simulink model "VFD3"  (R2020a)
settings: Solver=VariableStepAuto  StartTime=0.0  StopTime=100  RelTol=0.5e-3
libraries: fl_lib x51, nesl_utility x29, ee_lib x15, powerlib_meascontrol x2
settings Model: Creator=WASHINGTON  LastModifiedBy=WASHINGTON
settings SolverCC: MaxConsecutiveMinStep=100  AlgebraicLoopSolver=LineSearch

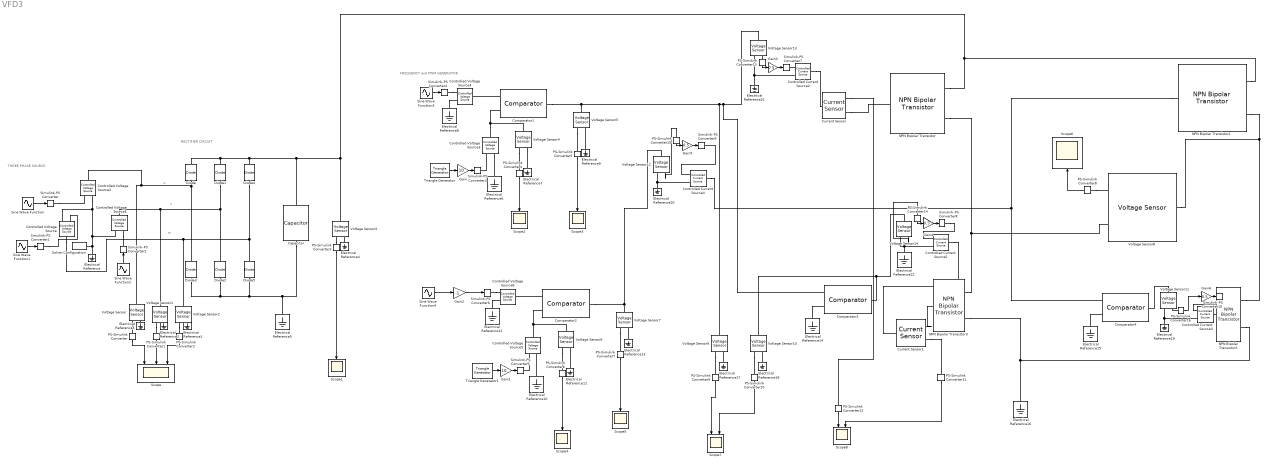
== system VFD3 ==
  note: FREQUENCY and PWM GENERATOR
  note: RECTIFIER CIRCUIT
  note: w
  note: v
  note: u
  note: THREE PHASE SOURCE
  Capacitor : ee_lib/Passive/Capacitor  cap_option=0  c=1 mF  Cvec=[1e-05, 1e-06] F  Vvec=[0, 10] V  CV_table_symmetry=1  f_vec=[1, 10] kHz  DFext_vec=[.8, 1.2]  C_tol=5  enable_C_tol=0  tol_distribution=1  nSigma=4  r=1e-6 Ohm  g=0 1/Ohm  averaging_period=0 s  enable_operating_limits=0  operating_limit_action=2  max_working_voltage_range=[-25, 25] V  power_rating=1 W  enable_faults=0  fault_action=1  Cscale_faulted=100  R_faulted=1e-3 Ohm  G_faulted=0 1/Ohm  tau_fault=1e-3 s  enable_temporal_fault=0  t_fault=1 s  enable_behavioral_fault=0  max_permissible_voltage_range=[-100, 100] V  t_fail_on_voltage=1 s  i_specify=off  i_priority=None  i=0 A  i_nominal_specify=off  i_nominal_unit=A  i_nominal_value=1  v_specify=off  v_priority=None  v=0 V  v_nominal_specify=off  v_nominal_unit=V  v_nominal_value=1  vc_specify=off  vc_priority=High  vc=0 V  vc_nominal_specify=off  vc_nominal_unit=V  vc_nominal_value=1
  Comparator{1..4} (4 alike) : ee_lib/Integrated Circuits/Comparator  V_OS=5 mV  V_OL=0 V  V_OH=10 V  C_IN=0 pF  R_OUT=50 Ohm  Delay=0 s
      settings: SourceProductBaseCode=PS  InternalSimscapePortConfiguration="{\"Bottom\":[],\"Left\":[{\"id\":\"p\",\"label\":\"+\",\"type\":\"foundation.electrical.electrical\"},{\"id\":\"n\",\"label\":\"-\",\"type\":\"foundation.electrical.electrical\"}],\"Right\":[{\"id\":\"J\",\"label\":\"\",\"type\":\"foundation.electrical.electrical\"}],\"Top\":[]}"
  Controlled Current Source{2..5} (4 alike) : fl_lib/Electrical/Electrical Sources/Controlled Current Source
  Controlled Voltage Source{,1..6} (7 alike) : fl_lib/Electrical/Electrical Sources/Controlled Voltage Source
  Current Sensor : fl_lib/Electrical/Electrical Sensors/Current Sensor
  Current Sensor1 : fl_lib/Electrical/Electrical Sensors/Current Sensor
  Diode{,1..5} (6 alike) : ee_lib/Semiconductors & Converters/Diode  ModelType=ee.enum.diode.modelType.pwl  Vf=0.6 V  Ron=0.3 Ohm  Goff=1e-8 S  prmExp=ee.enum.diode.expParam.useTwo  I12=[.0137, .545] A  V12=[.6, .7] V  IS=1e-12 A  ec=1  I1=0.0137 A  V1=0.6 V  RS=0 Ohm  Tmeas=25 degC  N_series=1  N_parallel=1  Rz=0.3 Ohm  BV=inf V  C_param=ee.enum.diode.capParam.fixed  CJ=5 pF  CJ0=5 pF  VJ=1 V  Mgrad=0.5  Vvec=[.1, 10, 100] V  Cvec=[3.5, 1, .4] pF  FC=0.5  Q_param=ee.enum.diode.recoveryParam.off  iRM=-7.15 A  iF=4 A  didt=-750 A/us  trr_factor=3  trr=115 ns  Qrr=1500 s*uA  TT=50 ns  tau=100 ns  T_param=ee.enum.diode.temperatureParam.off  IS_T2=1.25e-7 A  I1_T2=0.245 A  V1_T2=0.5 V  Tmeas2=125 degC  EG_param=ee.enum.diode.egapParam.material_si  EG=1.11 eV  XTI_param=ee.enum.diode.xtiParam.pn  XTI=3  dBVdT=0 V/K  Tdevice=25 degC  i_specify=off  i_priority=None  i=0 A  i_nominal_specify=off  i_nominal_unit=A  i_nominal_value=1  v_specify=off  v_priority=None  v=0 V  v_nominal_specify=off  v_nominal_unit=V  v_nominal_value=1  i_capacitor_specify=off  i_capacitor_priority=None  i_capacitor=0 A  i_capacitor_nominal_specify=off  i_capacitor_nominal_unit=A  i_capacitor_nominal_value=1  v_capacitor_specify=off  v_capacitor_priority=None  v_capacitor=0 V  v_capacitor_nominal_specify=off  v_capacitor_nominal_unit=V  v_capacitor_nominal_value=1  power_dissipated_specify=off  power_dissipated_priority=None  power_dissipated=0 W  power_dissipated_nominal_specify=off  power_dissipated_nominal_unit=W  power_dissipated_nominal_value=1  thermal_network_parameterization=ee.enum.thermalNetworkTopology.cauer  Rth=[0, 10] K/W  Rth_Foster=[4, 6] K/W  thermal_mass_parameterization=ee.enum.thermalNetwork.timeconstant  thermal_mass=[0, 1] J/K  thermal_mass_Foster=[1.5, 3] J/K  thermal_time_constant=[0, 10] s  thermal_time_constant_Foster=[6, 18] s  thermal_mass_initial_temperatures=[25, 25] degC
  Electrical Reference{,1..22} (23 alike) : fl_lib/Electrical/Electrical Elements/Electrical Reference
      settings: SourceProductBaseCode=MT,SS
  Gain : Gain  Gain=10
  Gain1 : Gain  Gain=10
  Gain2 : Gain  Gain=-1
  Gain{3..6} (4 alike) : Gain  Gain=0.5
  NPN Bipolar Transistor{,1..3} (4 alike) : ee_lib/Semiconductors & Converters/NPN Bipolar Transistor  parameterization=1  prmDatasheet=1  prmEquCoeff=1  BF=100  IS=1e-14 A  VAF=200 V  hfe=100  hoe=50e-6 1/Ohm  Ic_h=1 mA  Vce_h=5 V  V1=0.55 V  I1=0.5 mA  BR=1  Tmeas=25 degC  RC=0.01 Ohm  RE=1e-4 Ohm  RB=1 Ohm  C_BC=5 pF  C_BE=5 pF  TF=0 us  TR=0 us  hfe_T2=125  XTB=0  V1_T2=0.45 V  I1_T2=0.5 mA  Tmeas2=125 degC  EG=1.11 eV  XTI=3  ec=1  TdeviceDatasheet=25 degC  TdeviceEquCoeff=25 degC  thermal_network_parameterization=ee.enum.thermalNetworkTopology.cauer  Rth=[0, 10] K/W  Rth_Foster=[4, 6] K/W  thermal_mass_parameterization=ee.enum.thermalNetwork.timeconstant  thermal_mass=[0, 1] J/K  thermal_mass_Foster=[1.5, 3] J/K  thermal_time_constant=[0, 10] s  thermal_time_constant_Foster=[6, 18] s  thermal_mass_initial_temperatures=[25, 25] degC
  PS-Simulink Converter{,1..16} (17 alike) : nesl_utility/PS-Simulink Converter  PhysicalDomain=network_engine_domain  SubClassName=ps_output  LeftPortType=input  RightPortType=output  PseudoPeriodic=off  Frequencies=[]  Unit=inherit  AffineConversion=off
  Scope : Scope  NumInputPorts=3
  Scope{1..6} (6 alike) : Scope
  Scope7 : Scope  NumInputPorts=2
  Scope8 : Scope  NumInputPorts=2
  Simulink-PS Converter{,1..10} (11 alike) : nesl_utility/Simulink-PS Converter  PhysicalDomain=network_engine_domain  SubClassName=ps_input  LeftPortType=input  RightPortType=output  PseudoPeriodic=off  Frequencies=[]  NoiseDistribution=none  NoiseParameters=[]  Unit=1  AffineConversion=off  FilteringAndDerivatives=provide  SimscapeFilterOrder=1  InputFilterTimeConstant=0.001  UdotUserProvided=0
  Sine Wave Function : Sin  Amplitude=10  SampleTime=0
  Sine Wave Function1 : Sin  Amplitude=10  Phase=(2/3)*3.1415926535897932384626433832795028841971  SampleTime=0
  Sine Wave Function2 : Sin  Amplitude=10  Phase=(4/3)*3.1415926535897932384626433832795028841971  SampleTime=0
  Sine Wave Function3 : Sin  Amplitude=10  SampleTime=0
  Sine Wave Function4 : Sin  Amplitude=10  SampleTime=0
  Solver Configuration : nesl_utility/Solver Configuration  PhysicalDomain=network_engine_domain  SubClassName=solver  LeftPortType=input  RightPortType=generic  Tones=[]  Harmonics=[]  SimulateNoise=off  Profile=off  UseLocalSampling=off  EnableSwitchedLinearOptims=on  FrequencyDomain=off  UseCCode=off  RelTol=0.001  AbsTol=1e-06  MinStep=1e-09  ToWorkspace=off  RevertToSquareIcSolve=off  NumHomotopyIterations=100  PhasorMode=off  PhasorModeNumHarmonics=1  DoDC=off  ResidualTolerance=1e-09  UseLocalSolver=off  LocalSolverChoice=NE_BACKWARD_EULER_ADVANCER  LocalSolverSampleTime=0.001  DoFixedCost=off  MaxNonlinIter=3  MaxModeIter=2  LinearAlgebra=auto  EquationFormulation=NE_TIME_EF  DelaysMemoryBudget=1024  AutomaticFiltering=on  FilteringTimeConstant=0.001  PartitionStorageMethod=AS_NEEDED  PartitionMemoryBudget=1024  PartitionMethod=ROBUST
  Triangle Generator : powerlib_meascontrol/Pulse & Signal Generators/Triangle Generator  Freq=1  Phase=90  Ts=0
  Triangle Generator1 : powerlib_meascontrol/Pulse & Signal Generators/Triangle Generator  Freq=1  Phase=90  Ts=0
  Voltage Sensor{,1..14} (15 alike) : fl_lib/Electrical/Electrical Sensors/Voltage Sensor
  wires:
  Sine Wave Function/1 -> Simulink-PS Converter/1
  Sine Wave Function1/1 -> Simulink-PS Converter1/1
  Sine Wave Function2/1 -> Simulink-PS Converter2/1
  PS-Simulink Converter/1 -> Scope/1
  PS-Simulink Converter1/1 -> Scope/2
  PS-Simulink Converter2/1 -> Scope/3
  PS-Simulink Converter3/1 -> Scope1/1
  PS-Simulink Converter4/1 -> Scope2/1
  Triangle Generator/1 -> Gain/1
  Gain/1 -> Simulink-PS Converter3/1
  Sine Wave Function3/1 -> Simulink-PS Converter4/1
  PS-Simulink Converter5/1 -> Scope3/1
  PS-Simulink Converter7/1 -> Scope5/1
  Triangle Generator1/1 -> Gain1/1
  Gain1/1 -> Simulink-PS Converter5/1
  PS-Simulink Converter6/1 -> Scope4/1
  Gain2/1 -> Simulink-PS Converter6/1
  Sine Wave Function4/1 -> Gain2/1
  PS-Simulink Converter8/1 -> Scope6/1
  PS-Simulink Converter9/1 -> Scope7/1
  PS-Simulink Converter10/1 -> Scope7/2
  PS-Simulink Converter12/1 -> Scope8/1
  PS-Simulink Converter11/1 -> Scope8/2
  PS-Simulink Converter13/1 -> Gain3/1
  Gain3/1 -> Simulink-PS Converter7/1
  PS-Simulink Converter16/1 -> Gain6/1
  Gain6/1 -> Simulink-PS Converter10/1
  PS-Simulink Converter14/1 -> Gain4/1
  Gain4/1 -> Simulink-PS Converter8/1
  PS-Simulink Converter15/1 -> Gain5/1
  Gain5/1 -> Simulink-PS Converter9/1
  connections:
  Controlled Voltage Source2/RConn2 -- Solver Configuration/RConn1 -- Electrical Reference/LConn1 -- Controlled Voltage Source1/RConn2 -- Controlled Voltage Source/RConn2
  Controlled Voltage Source1/RConn1 -- Simulink-PS Converter2/RConn1
  Simulink-PS Converter1/RConn1 -- Controlled Voltage Source/RConn1
  Simulink-PS Converter/RConn1 -- Controlled Voltage Source2/RConn1
  Diode/LConn1 -- Voltage Sensor/LConn1 -- Controlled Voltage Source2/LConn1 -- Diode3/RConn1
  Diode1/LConn1 -- Controlled Voltage Source1/LConn1 -- Voltage Sensor1/LConn1 -- Diode2/RConn1
  Diode4/LConn1 -- Voltage Sensor2/LConn1 -- Controlled Voltage Source/LConn1 -- Diode5/RConn1
  Diode3/LConn1 -- Diode2/LConn1 -- Capacitor/RConn1 -- Electrical Reference5/LConn1 -- Diode5/LConn1
  Voltage Sensor/RConn1 -- PS-Simulink Converter/LConn1
  Voltage Sensor1/RConn1 -- PS-Simulink Converter1/LConn1
  Voltage Sensor2/RConn1 -- PS-Simulink Converter2/LConn1
  Electrical Reference1/LConn1 -- Voltage Sensor2/RConn2
  Voltage Sensor3/RConn1 -- PS-Simulink Converter3/LConn1
  Electrical Reference4/LConn1 -- Voltage Sensor3/RConn2
  Electrical Reference3/LConn1 -- Voltage Sensor/RConn2
  Electrical Reference2/LConn1 -- Voltage Sensor1/RConn2
  Simulink-PS Converter3/RConn1 -- Controlled Voltage Source3/RConn1
  Controlled Voltage Source3/LConn1 -- Comparator1/LConn1 -- Voltage Sensor4/LConn1
  Electrical Reference6/LConn1 -- Controlled Voltage Source3/RConn2
  Voltage Sensor4/RConn1 -- PS-Simulink Converter4/LConn1
  Electrical Reference7/LConn1 -- Voltage Sensor4/RConn2
  Simulink-PS Converter4/RConn1 -- Controlled Voltage Source4/RConn1
  Comparator1/LConn2 -- Controlled Voltage Source4/LConn1
  Electrical Reference8/LConn1 -- Controlled Voltage Source4/RConn2
  Electrical Reference9/LConn1 -- Voltage Sensor5/RConn2
  Voltage Sensor5/RConn1 -- PS-Simulink Converter5/LConn1
  Controlled Voltage Source5/LConn1 -- Comparator2/LConn1 -- Voltage Sensor6/LConn1
  Electrical Reference10/LConn1 -- Controlled Voltage Source5/RConn2
  Voltage Sensor7/RConn1 -- PS-Simulink Converter7/LConn1
  Comparator2/LConn2 -- Controlled Voltage Source6/LConn1
  Electrical Reference12/LConn1 -- Controlled Voltage Source6/RConn2
  Simulink-PS Converter6/RConn1 -- Controlled Voltage Source6/RConn1
  Comparator2/RConn1 -- Voltage Sensor12/LConn1 -- Voltage Sensor7/LConn1
  Simulink-PS Converter5/RConn1 -- Controlled Voltage Source5/RConn1
  Voltage Sensor6/RConn1 -- PS-Simulink Converter6/LConn1
  Electrical Reference11/LConn1 -- Voltage Sensor6/RConn2
  Electrical Reference13/LConn1 -- Voltage Sensor7/RConn2
  Voltage Sensor8/RConn2 -- NPN Bipolar Transistor3/RConn1 -- NPN Bipolar Transistor/RConn2
  Voltage Sensor8/LConn1 -- NPN Bipolar Transistor2/RConn1 -- NPN Bipolar Transistor1/RConn2
  Diode/RConn1 -- Diode1/RConn1 -- Capacitor/LConn1 -- Voltage Sensor3/LConn1 -- NPN Bipolar Transistor1/RConn1 -- NPN Bipolar Transistor/RConn1 -- Diode4/RConn1
  Electrical Reference16/LConn1 -- NPN Bipolar Transistor2/RConn2 -- NPN Bipolar Transistor3/RConn2
  PS-Simulink Converter8/LConn1 -- Voltage Sensor8/RConn1
  Comparator1/RConn1 -- Voltage Sensor5/LConn1 -- Comparator3/LConn2 -- Voltage Sensor13/LConn1 -- Voltage Sensor9/LConn1
  Electrical Reference17/LConn1 -- Voltage Sensor9/RConn2
  Voltage Sensor9/RConn1 -- PS-Simulink Converter9/LConn1
  Voltage Sensor10/RConn1 -- PS-Simulink Converter10/LConn1
  Electrical Reference18/LConn1 -- Voltage Sensor10/RConn2
  Comparator3/RConn1 -- Voltage Sensor14/LConn1 -- Voltage Sensor10/LConn1
  Electrical Reference14/LConn1 -- Comparator3/LConn1
  Electrical Reference15/LConn1 -- Comparator4/LConn1
  Current Sensor/RConn2 -- NPN Bipolar Transistor/LConn1
  Current Sensor1/RConn2 -- NPN Bipolar Transistor3/LConn1
  Current Sensor1/RConn1 -- PS-Simulink Converter11/LConn1
  Current Sensor/RConn1 -- PS-Simulink Converter12/LConn1
  PS-Simulink Converter16/LConn1 -- Voltage Sensor11/RConn1
  Electrical Reference19/LConn1 -- Voltage Sensor11/RConn2 -- Controlled Current Source3/RConn2
  Controlled Current Source3/LConn1 -- NPN Bipolar Transistor2/LConn1
  Comparator4/RConn1 -- Voltage Sensor11/LConn1
  Electrical Reference20/LConn1 -- Voltage Sensor12/RConn2 -- Controlled Current Source4/RConn2
  Voltage Sensor12/RConn1 -- PS-Simulink Converter15/LConn1
  NPN Bipolar Transistor1/LConn1 -- Controlled Current Source4/LConn1 -- Comparator4/LConn2
  Electrical Reference21/LConn1 -- Controlled Current Source2/RConn2 -- Voltage Sensor13/RConn2
  Controlled Current Source2/LConn1 -- Current Sensor/LConn1
  Controlled Current Source5/RConn2 -- Electrical Reference22/LConn1 -- Voltage Sensor14/RConn2
  Controlled Current Source5/LConn1 -- Current Sensor1/LConn1
  Voltage Sensor14/RConn1 -- PS-Simulink Converter14/LConn1
  Voltage Sensor13/RConn1 -- PS-Simulink Converter13/LConn1
  Simulink-PS Converter7/RConn1 -- Controlled Current Source2/RConn1
  Simulink-PS Converter10/RConn1 -- Controlled Current Source3/RConn1
  Simulink-PS Converter8/RConn1 -- Controlled Current Source5/RConn1
  Controlled Current Source4/RConn1 -- Simulink-PS Converter9/RConn1
